simulink model "PVtestsiteeight"  (Simulink 10.1)
settings: Solver=FixedStepDiscrete  StartTime=0.0  StopTime=inf  FixedStep=Ts  RelTol=1e-3
PreLoadFcn:
  | init_DCDCDCAC_new
InitFcn:
  | init_DCDCDCAC_new
undefined symbols (not defined in the file or in its folder): D1, Delta, I, Left, Right, type, V
libraries: powerlib x174, powerlib_meascontrol x3, ssn_lib x2, artemis x1
(part 3 of 3)

== system PVtestsiteeight/SS_Grid/733 ==
  Three-Phase V-I Measurement : powerlib/Measurements/Three-Phase V-I Measurement  VoltageMeasurement=phase-to-ground  SetLabelV=off  LabelV=Vabc  Vpu=off  VpuLL=off  CurrentMeasurement=yes  SetLabelI=off  LabelI=Iabc  Ipu=off  Pbase=100e6  Vbase=500e3  OutputType=Complex  PhasorSimulation=off  PSBequivalent=0
  Conn1 : PMIOPort  Side=Left
  Conn2 : PMIOPort  Port=2  Side=Left
  Conn3 : PMIOPort  Port=3  Side=Right
  Conn4 : PMIOPort  Port=4  Side=Right
  Conn5 : PMIOPort  Port=5  Side=Left
  Conn6 : PMIOPort  Port=6  Side=Right
  tag scope: I_733=global, V_733=global
  wires:
  Three-Phase V-I Measurement/1 -> [V_733]
  Three-Phase V-I Measurement/2 -> [I_733]
  connections:
  Conn1/RConn1 -- Three-Phase V-I Measurement/LConn1
  Conn2/RConn1 -- Three-Phase V-I Measurement/LConn2
  Conn3/RConn1 -- Three-Phase V-I Measurement/RConn1
  Conn4/RConn1 -- Three-Phase V-I Measurement/RConn2
  Conn5/RConn1 -- Three-Phase V-I Measurement/LConn3
  Conn6/RConn1 -- Three-Phase V-I Measurement/RConn3

== system PVtestsiteeight/SS_Grid/733 - 734 Conf 723 ==
  Pi Section Line : powerlib/Elements/Pi Section Line  LConnTagsString=__new0  RConnTagsString=__new0  Frequency=60  Resistance=0.803807  Inductance=0.0011064  Capacitance=1.23355e-07  Length=D  PiSections=1  Measurements=None
      settings: AttributesFormatString=\n  SourceProductBaseCode=PS
  Pi Section Line1 : powerlib/Elements/Pi Section Line  LConnTagsString=__new0  RConnTagsString=__new0  Frequency=60  Resistance=0.80915157  Inductance=0.00104267  Capacitance=1.233552e-07  Length=D  PiSections=1  Measurements=None
      settings: AttributesFormatString=\n  SourceProductBaseCode=PS
  Pi Section Line2 : powerlib/Elements/Pi Section Line  LConnTagsString=__new0  RConnTagsString=__new0  Frequency=60  Resistance=0.8038077  Inductance=0.0011064  Capacitance=1.23355e-07  Length=D  PiSections=1  Measurements=None
      settings: AttributesFormatString=\n  SourceProductBaseCode=PS
  a : PMIOPort  Side=Left
  A : PMIOPort  Port=2  Side=Right
  b : PMIOPort  Port=3  Side=Left
  B : PMIOPort  Port=4  Side=Right
  c : PMIOPort  Port=5  Side=Left
  C : PMIOPort  Port=6  Side=Right
  connections:
  C/RConn1 -- Pi Section Line2/RConn1
  c/RConn1 -- Pi Section Line2/LConn1
  B/RConn1 -- Pi Section Line1/RConn1
  b/RConn1 -- Pi Section Line1/LConn1
  A/RConn1 -- Pi Section Line/RConn1
  a/RConn1 -- Pi Section Line/LConn1

== system PVtestsiteeight/SS_Grid/734 ==
  Three-Phase V-I Measurement : powerlib/Measurements/Three-Phase V-I Measurement  VoltageMeasurement=phase-to-ground  SetLabelV=off  LabelV=Vabc  Vpu=off  VpuLL=off  CurrentMeasurement=yes  SetLabelI=off  LabelI=Iabc  Ipu=off  Pbase=100e6  Vbase=500e3  OutputType=Complex  PhasorSimulation=off  PSBequivalent=0
  Conn1 : PMIOPort  Side=Left
  Conn2 : PMIOPort  Port=2  Side=Left
  Conn3 : PMIOPort  Port=3  Side=Right
  Conn4 : PMIOPort  Port=4  Side=Right
  Conn5 : PMIOPort  Port=5  Side=Left
  Conn6 : PMIOPort  Port=6  Side=Right
  tag scope: I_734=global, V_734=global
  wires:
  Three-Phase V-I Measurement/2 -> [I_734]
  Three-Phase V-I Measurement/1 -> [V_734]
  connections:
  Conn6/RConn1 -- Three-Phase V-I Measurement/RConn3
  Conn5/RConn1 -- Three-Phase V-I Measurement/LConn3
  Conn4/RConn1 -- Three-Phase V-I Measurement/RConn2
  Conn3/RConn1 -- Three-Phase V-I Measurement/RConn1
  Conn2/RConn1 -- Three-Phase V-I Measurement/LConn2
  Conn1/RConn1 -- Three-Phase V-I Measurement/LConn1

== system PVtestsiteeight/SS_Grid/734 - 710 config 724  ==
  Pi Section Line : powerlib/Elements/Pi Section Line  LConnTagsString=__new0  RConnTagsString=__new0  Frequency=60  Resistance=1.3019001  Inductance=0.0012787  Capacitance=9.93038e-08  Length=D  PiSections=1  Measurements=None
      settings: AttributesFormatString=\n  SourceProductBaseCode=PS
  Pi Section Line1 : powerlib/Elements/Pi Section Line  LConnTagsString=__new0  RConnTagsString=__new0  Frequency=60  Resistance=1.309108  Inductance=0.001219369  Capacitance=9.9303e-08  Length=D  PiSections=1  Measurements=None
      settings: AttributesFormatString=\n  SourceProductBaseCode=PS
  Pi Section Line2 : powerlib/Elements/Pi Section Line  LConnTagsString=__new0  RConnTagsString=__new0  Frequency=60  Resistance=1.3019001  Inductance=0.0012787  Capacitance=9.93038e-08  Length=D  PiSections=1  Measurements=None
      settings: AttributesFormatString=\n  SourceProductBaseCode=PS
  a : PMIOPort  Side=Left
  A : PMIOPort  Port=2  Side=Right
  b : PMIOPort  Port=3  Side=Left
  B : PMIOPort  Port=4  Side=Right
  c : PMIOPort  Port=5  Side=Left
  C : PMIOPort  Port=6  Side=Right
  connections:
  a/RConn1 -- Pi Section Line/LConn1
  A/RConn1 -- Pi Section Line/RConn1
  b/RConn1 -- Pi Section Line1/LConn1
  B/RConn1 -- Pi Section Line1/RConn1
  c/RConn1 -- Pi Section Line2/LConn1
  C/RConn1 -- Pi Section Line2/RConn1

== system PVtestsiteeight/SS_Grid/734 - 737 Conf 723  ==
  Pi Section Line : powerlib/Elements/Pi Section Line  LConnTagsString=__new0  RConnTagsString=__new0  Frequency=60  Resistance=0.803807  Inductance=0.0011064  Capacitance=1.23355e-07  Length=D  PiSections=1  Measurements=None
      settings: AttributesFormatString=\n  SourceProductBaseCode=PS
  Pi Section Line1 : powerlib/Elements/Pi Section Line  LConnTagsString=__new0  RConnTagsString=__new0  Frequency=60  Resistance=0.80915157  Inductance=0.00104267  Capacitance=1.233552e-07  Length=D  PiSections=1  Measurements=None
      settings: AttributesFormatString=\n  SourceProductBaseCode=PS
  Pi Section Line2 : powerlib/Elements/Pi Section Line  LConnTagsString=__new0  RConnTagsString=__new0  Frequency=60  Resistance=0.8038077  Inductance=0.0011064  Capacitance=1.23355e-07  Length=D  PiSections=1  Measurements=None
      settings: AttributesFormatString=\n  SourceProductBaseCode=PS
  a : PMIOPort  Side=Left
  A : PMIOPort  Port=2  Side=Right
  b : PMIOPort  Port=3  Side=Left
  B : PMIOPort  Port=4  Side=Right
  c : PMIOPort  Port=5  Side=Left
  C : PMIOPort  Port=6  Side=Right
  connections:
  a/RConn1 -- Pi Section Line/LConn1
  A/RConn1 -- Pi Section Line/RConn1
  b/RConn1 -- Pi Section Line1/LConn1
  B/RConn1 -- Pi Section Line1/RConn1
  c/RConn1 -- Pi Section Line2/LConn1
  C/RConn1 -- Pi Section Line2/RConn1

== system PVtestsiteeight/SS_Grid/735 ==
  Three-Phase V-I Measurement : powerlib/Measurements/Three-Phase V-I Measurement  VoltageMeasurement=phase-to-ground  SetLabelV=off  LabelV=Vabc  Vpu=off  VpuLL=off  CurrentMeasurement=yes  SetLabelI=off  LabelI=Iabc  Ipu=off  Pbase=100e6  Vbase=500e3  OutputType=Complex  PhasorSimulation=off  PSBequivalent=0
  Conn1 : PMIOPort  Side=Left
  Conn2 : PMIOPort  Port=2  Side=Left
  Conn3 : PMIOPort  Port=3  Side=Right
  Conn4 : PMIOPort  Port=4  Side=Right
  Conn5 : PMIOPort  Port=5  Side=Left
  Conn6 : PMIOPort  Port=6  Side=Right
  tag scope: I_735=global, V_735=global
  wires:
  Three-Phase V-I Measurement/1 -> [V_735]
  Three-Phase V-I Measurement/2 -> [I_735]
  connections:
  Conn1/RConn1 -- Three-Phase V-I Measurement/LConn1
  Conn2/RConn1 -- Three-Phase V-I Measurement/LConn2
  Conn3/RConn1 -- Three-Phase V-I Measurement/RConn1
  Conn4/RConn1 -- Three-Phase V-I Measurement/RConn2
  Conn5/RConn1 -- Three-Phase V-I Measurement/LConn3
  Conn6/RConn1 -- Three-Phase V-I Measurement/RConn3

== system PVtestsiteeight/SS_Grid/736 ==
  Three-Phase V-I Measurement : powerlib/Measurements/Three-Phase V-I Measurement  VoltageMeasurement=phase-to-ground  SetLabelV=off  LabelV=Vabc  Vpu=off  VpuLL=off  CurrentMeasurement=yes  SetLabelI=off  LabelI=Iabc  Ipu=off  Pbase=100e6  Vbase=500e3  OutputType=Complex  PhasorSimulation=off  PSBequivalent=0
  Conn1 : PMIOPort  Side=Left
  Conn2 : PMIOPort  Port=2  Side=Left
  Conn3 : PMIOPort  Port=3  Side=Right
  Conn4 : PMIOPort  Port=4  Side=Right
  Conn5 : PMIOPort  Port=5  Side=Left
  Conn6 : PMIOPort  Port=6  Side=Right
  tag scope: I_736=global, V_736=global
  wires:
  Three-Phase V-I Measurement/2 -> [I_736]
  Three-Phase V-I Measurement/1 -> [V_736]
  connections:
  Conn6/RConn1 -- Three-Phase V-I Measurement/RConn3
  Conn5/RConn1 -- Three-Phase V-I Measurement/LConn3
  Conn4/RConn1 -- Three-Phase V-I Measurement/RConn2
  Conn3/RConn1 -- Three-Phase V-I Measurement/RConn1
  Conn2/RConn1 -- Three-Phase V-I Measurement/LConn2
  Conn1/RConn1 -- Three-Phase V-I Measurement/LConn1

== system PVtestsiteeight/SS_Grid/737 ==
  Three-Phase V-I Measurement : powerlib/Measurements/Three-Phase V-I Measurement  VoltageMeasurement=phase-to-ground  SetLabelV=off  LabelV=Vabc  Vpu=off  VpuLL=off  CurrentMeasurement=yes  SetLabelI=off  LabelI=Iabc  Ipu=off  Pbase=100e6  Vbase=500e3  OutputType=Complex  PhasorSimulation=off  PSBequivalent=0
  Conn1 : PMIOPort  Side=Left
  Conn2 : PMIOPort  Port=2  Side=Left
  Conn3 : PMIOPort  Port=3  Side=Right
  Conn4 : PMIOPort  Port=4  Side=Right
  Conn5 : PMIOPort  Port=5  Side=Left
  Conn6 : PMIOPort  Port=6  Side=Right
  tag scope: I_737=global, V_737=global
  wires:
  Three-Phase V-I Measurement/1 -> [V_737]
  Three-Phase V-I Measurement/2 -> [I_737]
  connections:
  Conn1/RConn1 -- Three-Phase V-I Measurement/LConn1
  Conn2/RConn1 -- Three-Phase V-I Measurement/LConn2
  Conn3/RConn1 -- Three-Phase V-I Measurement/RConn1
  Conn4/RConn1 -- Three-Phase V-I Measurement/RConn2
  Conn5/RConn1 -- Three-Phase V-I Measurement/LConn3
  Conn6/RConn1 -- Three-Phase V-I Measurement/RConn3

== system PVtestsiteeight/SS_Grid/737 - 738 Conf 723  ==
  Pi Section Line : powerlib/Elements/Pi Section Line  LConnTagsString=__new0  RConnTagsString=__new0  Frequency=60  Resistance=0.803807  Inductance=0.0011064  Capacitance=1.23355e-07  Length=D  PiSections=1  Measurements=None
      settings: AttributesFormatString=\n  SourceProductBaseCode=PS
  Pi Section Line1 : powerlib/Elements/Pi Section Line  LConnTagsString=__new0  RConnTagsString=__new0  Frequency=60  Resistance=0.80915157  Inductance=0.00104267  Capacitance=1.233552e-07  Length=D  PiSections=1  Measurements=None
      settings: AttributesFormatString=\n  SourceProductBaseCode=PS
  Pi Section Line2 : powerlib/Elements/Pi Section Line  LConnTagsString=__new0  RConnTagsString=__new0  Frequency=60  Resistance=0.8038077  Inductance=0.0011064  Capacitance=1.23355e-07  Length=D  PiSections=1  Measurements=None
      settings: AttributesFormatString=\n  SourceProductBaseCode=PS
  a : PMIOPort  Side=Left
  A : PMIOPort  Port=2  Side=Right
  b : PMIOPort  Port=3  Side=Left
  B : PMIOPort  Port=4  Side=Right
  c : PMIOPort  Port=5  Side=Left
  C : PMIOPort  Port=6  Side=Right
  connections:
  C/RConn1 -- Pi Section Line2/RConn1
  c/RConn1 -- Pi Section Line2/LConn1
  B/RConn1 -- Pi Section Line1/RConn1
  b/RConn1 -- Pi Section Line1/LConn1
  A/RConn1 -- Pi Section Line/RConn1
  a/RConn1 -- Pi Section Line/LConn1

== system PVtestsiteeight/SS_Grid/738 ==
  Three-Phase V-I Measurement : powerlib/Measurements/Three-Phase V-I Measurement  VoltageMeasurement=phase-to-ground  SetLabelV=off  LabelV=Vabc  Vpu=off  VpuLL=off  CurrentMeasurement=yes  SetLabelI=off  LabelI=Iabc  Ipu=off  Pbase=100e6  Vbase=500e3  OutputType=Complex  PhasorSimulation=off  PSBequivalent=0
  Conn1 : PMIOPort  Side=Left
  Conn2 : PMIOPort  Port=2  Side=Left
  Conn3 : PMIOPort  Port=3  Side=Right
  Conn4 : PMIOPort  Port=4  Side=Right
  Conn5 : PMIOPort  Port=5  Side=Left
  Conn6 : PMIOPort  Port=6  Side=Right
  tag scope: I_738=global, V_738=global
  wires:
  Three-Phase V-I Measurement/2 -> [I_738]
  Three-Phase V-I Measurement/1 -> [V_738]
  connections:
  Conn6/RConn1 -- Three-Phase V-I Measurement/RConn3
  Conn5/RConn1 -- Three-Phase V-I Measurement/LConn3
  Conn4/RConn1 -- Three-Phase V-I Measurement/RConn2
  Conn3/RConn1 -- Three-Phase V-I Measurement/RConn1
  Conn2/RConn1 -- Three-Phase V-I Measurement/LConn2
  Conn1/RConn1 -- Three-Phase V-I Measurement/LConn1

== system PVtestsiteeight/SS_Grid/740 ==
  Three-Phase V-I Measurement : powerlib/Measurements/Three-Phase V-I Measurement  VoltageMeasurement=phase-to-ground  SetLabelV=off  LabelV=Vabc  Vpu=off  VpuLL=off  CurrentMeasurement=yes  SetLabelI=off  LabelI=Iabc  Ipu=off  Pbase=100e6  Vbase=500e3  OutputType=Complex  PhasorSimulation=off  PSBequivalent=0
  Conn1 : PMIOPort  Side=Left
  Conn2 : PMIOPort  Port=2  Side=Left
  Conn3 : PMIOPort  Port=3  Side=Right
  Conn4 : PMIOPort  Port=4  Side=Right
  Conn5 : PMIOPort  Port=5  Side=Left
  Conn6 : PMIOPort  Port=6  Side=Right
  tag scope: I_740=global, V_740=global
  wires:
  Three-Phase V-I Measurement/2 -> [I_740]
  Three-Phase V-I Measurement/1 -> [V_740]
  connections:
  Conn6/RConn1 -- Three-Phase V-I Measurement/RConn3
  Conn5/RConn1 -- Three-Phase V-I Measurement/LConn3
  Conn4/RConn1 -- Three-Phase V-I Measurement/RConn2
  Conn3/RConn1 -- Three-Phase V-I Measurement/RConn1
  Conn2/RConn1 -- Three-Phase V-I Measurement/LConn2
  Conn1/RConn1 -- Three-Phase V-I Measurement/LConn1

== system PVtestsiteeight/SS_Grid/741 ==
  Three-Phase V-I Measurement : powerlib/Measurements/Three-Phase V-I Measurement  VoltageMeasurement=phase-to-ground  SetLabelV=off  LabelV=Vabc  Vpu=off  VpuLL=off  CurrentMeasurement=yes  SetLabelI=off  LabelI=Iabc  Ipu=off  Pbase=100e6  Vbase=500e3  OutputType=Complex  PhasorSimulation=off  PSBequivalent=0
  Conn1 : PMIOPort  Side=Left
  Conn2 : PMIOPort  Port=2  Side=Left
  Conn3 : PMIOPort  Port=3  Side=Right
  Conn4 : PMIOPort  Port=4  Side=Right
  Conn5 : PMIOPort  Port=5  Side=Left
  Conn6 : PMIOPort  Port=6  Side=Right
  tag scope: I_741=global, V_741=global
  wires:
  Three-Phase V-I Measurement/2 -> [I_741]
  Three-Phase V-I Measurement/1 -> [V_741]
  connections:
  Conn6/RConn1 -- Three-Phase V-I Measurement/RConn3
  Conn5/RConn1 -- Three-Phase V-I Measurement/LConn3
  Conn4/RConn1 -- Three-Phase V-I Measurement/RConn2
  Conn3/RConn1 -- Three-Phase V-I Measurement/RConn1
  Conn2/RConn1 -- Three-Phase V-I Measurement/LConn2
  Conn1/RConn1 -- Three-Phase V-I Measurement/LConn1

== system PVtestsiteeight/SS_Grid/742 ==
  Three-Phase V-I Measurement : powerlib/Measurements/Three-Phase V-I Measurement  VoltageMeasurement=phase-to-ground  SetLabelV=off  LabelV=Vabc  Vpu=off  VpuLL=off  CurrentMeasurement=yes  SetLabelI=off  LabelI=Iabc  Ipu=off  Pbase=100e6  Vbase=500e3  OutputType=Complex  PhasorSimulation=off  PSBequivalent=0
  Conn1 : PMIOPort  Side=Left
  Conn2 : PMIOPort  Port=2  Side=Left
  Conn3 : PMIOPort  Port=3  Side=Right
  Conn4 : PMIOPort  Port=4  Side=Right
  Conn5 : PMIOPort  Port=5  Side=Left
  Conn6 : PMIOPort  Port=6  Side=Right
  tag scope: I_742=global, V_742=global
  wires:
  Three-Phase V-I Measurement/2 -> [I_742]
  Three-Phase V-I Measurement/1 -> [V_742]
  connections:
  Conn6/RConn1 -- Three-Phase V-I Measurement/RConn3
  Conn5/RConn1 -- Three-Phase V-I Measurement/LConn3
  Conn4/RConn1 -- Three-Phase V-I Measurement/RConn2
  Conn3/RConn1 -- Three-Phase V-I Measurement/RConn1
  Conn2/RConn1 -- Three-Phase V-I Measurement/LConn2
  Conn1/RConn1 -- Three-Phase V-I Measurement/LConn1

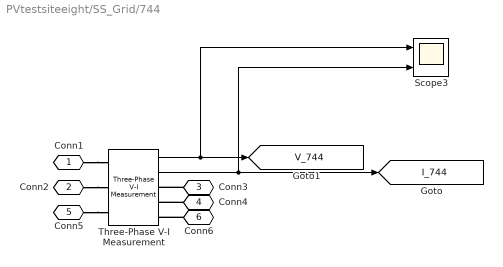
== system PVtestsiteeight/SS_Grid/744 ==
  Scope3 : Scope  NumInputPorts=2
  Three-Phase V-I Measurement : powerlib/Measurements/Three-Phase V-I Measurement  VoltageMeasurement=phase-to-ground  SetLabelV=off  LabelV=Vabc  Vpu=off  VpuLL=off  CurrentMeasurement=yes  SetLabelI=off  LabelI=Iabc  Ipu=off  Pbase=100e6  Vbase=500e3  OutputType=Complex  PhasorSimulation=off  PSBequivalent=0
  Conn1 : PMIOPort  Side=Left
  Conn2 : PMIOPort  Port=2  Side=Left
  Conn3 : PMIOPort  Port=3  Side=Right
  Conn4 : PMIOPort  Port=4  Side=Right
  Conn5 : PMIOPort  Port=5  Side=Left
  Conn6 : PMIOPort  Port=6  Side=Right
  tag scope: I_744=global, V_744=global
  wires:
  Three-Phase V-I Measurement/2 -> Scope3/2, [I_744]
  Three-Phase V-I Measurement/1 -> Scope3/1, [V_744]
  connections:
  Conn6/RConn1 -- Three-Phase V-I Measurement/RConn3
  Conn5/RConn1 -- Three-Phase V-I Measurement/LConn3
  Conn4/RConn1 -- Three-Phase V-I Measurement/RConn2
  Conn3/RConn1 -- Three-Phase V-I Measurement/RConn1
  Conn2/RConn1 -- Three-Phase V-I Measurement/LConn2
  Conn1/RConn1 -- Three-Phase V-I Measurement/LConn1

== system PVtestsiteeight/SS_Grid/744 - 728 config 724  ==
  Pi Section Line : powerlib/Elements/Pi Section Line  LConnTagsString=__new0  RConnTagsString=__new0  Frequency=60  Resistance=1.3019001  Inductance=0.0012787  Capacitance=9.93038e-08  Length=D  PiSections=1  Measurements=None
      settings: AttributesFormatString=\n  SourceProductBaseCode=PS
  Pi Section Line1 : powerlib/Elements/Pi Section Line  LConnTagsString=__new0  RConnTagsString=__new0  Frequency=60  Resistance=1.309108  Inductance=0.001219369  Capacitance=9.9303e-08  Length=D  PiSections=1  Measurements=None
      settings: AttributesFormatString=\n  SourceProductBaseCode=PS
  Pi Section Line2 : powerlib/Elements/Pi Section Line  LConnTagsString=__new0  RConnTagsString=__new0  Frequency=60  Resistance=1.3019001  Inductance=0.0012787  Capacitance=9.93038e-08  Length=D  PiSections=1  Measurements=None
      settings: AttributesFormatString=\n  SourceProductBaseCode=PS
  a : PMIOPort  Side=Left
  A : PMIOPort  Port=2  Side=Right
  b : PMIOPort  Port=3  Side=Left
  B : PMIOPort  Port=4  Side=Right
  c : PMIOPort  Port=5  Side=Left
  C : PMIOPort  Port=6  Side=Right
  connections:
  a/RConn1 -- Pi Section Line/LConn1
  A/RConn1 -- Pi Section Line/RConn1
  b/RConn1 -- Pi Section Line1/LConn1
  B/RConn1 -- Pi Section Line1/RConn1
  c/RConn1 -- Pi Section Line2/LConn1
  C/RConn1 -- Pi Section Line2/RConn1

== system PVtestsiteeight/SS_Grid/744 - 729 config 724  ==
  Pi Section Line : powerlib/Elements/Pi Section Line  LConnTagsString=__new0  RConnTagsString=__new0  Frequency=60  Resistance=1.3019001  Inductance=0.0012787  Capacitance=9.93038e-08  Length=D  PiSections=1  Measurements=None
      settings: AttributesFormatString=\n  SourceProductBaseCode=PS
  Pi Section Line1 : powerlib/Elements/Pi Section Line  LConnTagsString=__new0  RConnTagsString=__new0  Frequency=60  Resistance=1.309108  Inductance=0.001219369  Capacitance=9.9303e-08  Length=D  PiSections=1  Measurements=None
      settings: AttributesFormatString=\n  SourceProductBaseCode=PS
  Pi Section Line2 : powerlib/Elements/Pi Section Line  LConnTagsString=__new0  RConnTagsString=__new0  Frequency=60  Resistance=1.3019001  Inductance=0.0012787  Capacitance=9.93038e-08  Length=D  PiSections=1  Measurements=None
      settings: AttributesFormatString=\n  SourceProductBaseCode=PS
  a : PMIOPort  Side=Left
  A : PMIOPort  Port=2  Side=Right
  b : PMIOPort  Port=3  Side=Left
  B : PMIOPort  Port=4  Side=Right
  c : PMIOPort  Port=5  Side=Left
  C : PMIOPort  Port=6  Side=Right
  connections:
  C/RConn1 -- Pi Section Line2/RConn1
  c/RConn1 -- Pi Section Line2/LConn1
  B/RConn1 -- Pi Section Line1/RConn1
  b/RConn1 -- Pi Section Line1/LConn1
  A/RConn1 -- Pi Section Line/RConn1
  a/RConn1 -- Pi Section Line/LConn1

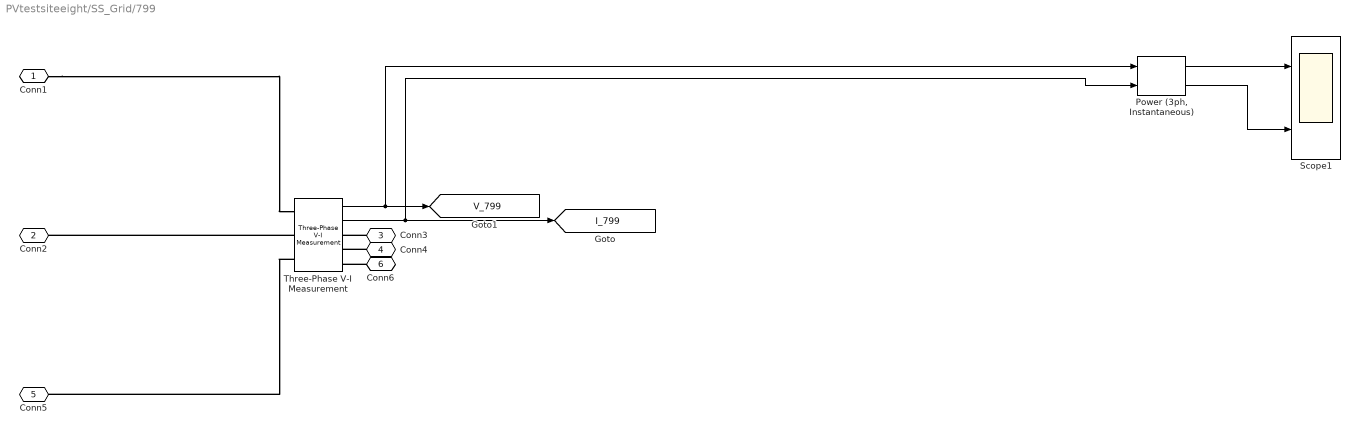
== system PVtestsiteeight/SS_Grid/799 ==
  "Power (3ph, Instantaneous)" : powerlib_meascontrol/Measurements/Power (3ph, Instantaneous)
  Scope1 : Scope  NumInputPorts=2
  Three-Phase V-I Measurement : powerlib/Measurements/Three-Phase V-I Measurement  VoltageMeasurement=phase-to-ground  SetLabelV=off  LabelV=Vabc  Vpu=off  VpuLL=off  CurrentMeasurement=yes  SetLabelI=off  LabelI=Iabc  Ipu=off  Pbase=100e6  Vbase=500e3  OutputType=Complex  PhasorSimulation=off  PSBequivalent=0
  Conn1 : PMIOPort  Side=Left
  Conn2 : PMIOPort  Port=2  Side=Left
  Conn3 : PMIOPort  Port=3  Side=Right
  Conn4 : PMIOPort  Port=4  Side=Right
  Conn5 : PMIOPort  Port=5  Side=Left
  Conn6 : PMIOPort  Port=6  Side=Right
  tag scope: I_799=global, V_799=global
  wires:
  Three-Phase V-I Measurement/2 -> "Power (3ph, Instantaneous)"/2, [I_799]
  Three-Phase V-I Measurement/1 -> "Power (3ph, Instantaneous)"/1, [V_799]
  "Power (3ph, Instantaneous)"/1 -> Scope1/1
  "Power (3ph, Instantaneous)"/2 -> Scope1/2
  connections:
  Conn1/RConn1 -- Three-Phase V-I Measurement/LConn1
  Three-Phase V-I Measurement/LConn2 -- Conn2/RConn1
  Conn3/RConn1 -- Three-Phase V-I Measurement/RConn1
  Conn4/RConn1 -- Three-Phase V-I Measurement/RConn2
  Three-Phase V-I Measurement/LConn3 -- Conn5/RConn1
  Conn6/RConn1 -- Three-Phase V-I Measurement/RConn3

== system PVtestsiteeight/SS_Grid/799 - 701 Configuration 721 ==
  Pi Section Line : powerlib/Elements/Pi Section Line  LConnTagsString=__new0  RConnTagsString=__new0  Frequency=60  Resistance=0.181813  Inductance=0.00032519  Capacitance=2.63375e-07  Length=D  PiSections=1  Measurements=None
      settings: AttributesFormatString=\n  SourceProductBaseCode=PS
  Pi Section Line1 : powerlib/Elements/Pi Section Line  LConnTagsString=__new0  RConnTagsString=__new0  Frequency=60  Resistance=0.164413  Inductance=0.000313166  Capacitance=2.633757e-07  Length=D  PiSections=1  Measurements=None
      settings: AttributesFormatString=\n  SourceProductBaseCode=PS
  Pi Section Line2 : powerlib/Elements/Pi Section Line  LConnTagsString=__new0  RConnTagsString=__new0  Frequency=60  Resistance=0.181813  Inductance=0.000325198  Capacitance=2.633757e-07  Length=D  PiSections=1  Measurements=None
      settings: AttributesFormatString=\n  SourceProductBaseCode=PS
  A : PMIOPort  Side=Left
  a : PMIOPort  Port=2  Side=Right
  B : PMIOPort  Port=3  Side=Left
  b : PMIOPort  Port=4  Side=Right
  C : PMIOPort  Port=5  Side=Left
  c : PMIOPort  Port=6  Side=Right
  connections:
  A/RConn1 -- Pi Section Line/LConn1
  a/RConn1 -- Pi Section Line/RConn1
  B/RConn1 -- Pi Section Line1/LConn1
  b/RConn1 -- Pi Section Line1/RConn1
  C/RConn1 -- Pi Section Line2/LConn1
  c/RConn1 -- Pi Section Line2/RConn1
